simulink model "Modelo_controlador_estados"  (R2021a)
settings: Solver=FixedStepAuto  StartTime=0.0  StopTime=6  FixedStep=0.001  RelTol=1e-3
libraries: simulink x1
settings Model: Creator=faust  LastModifiedBy=franc

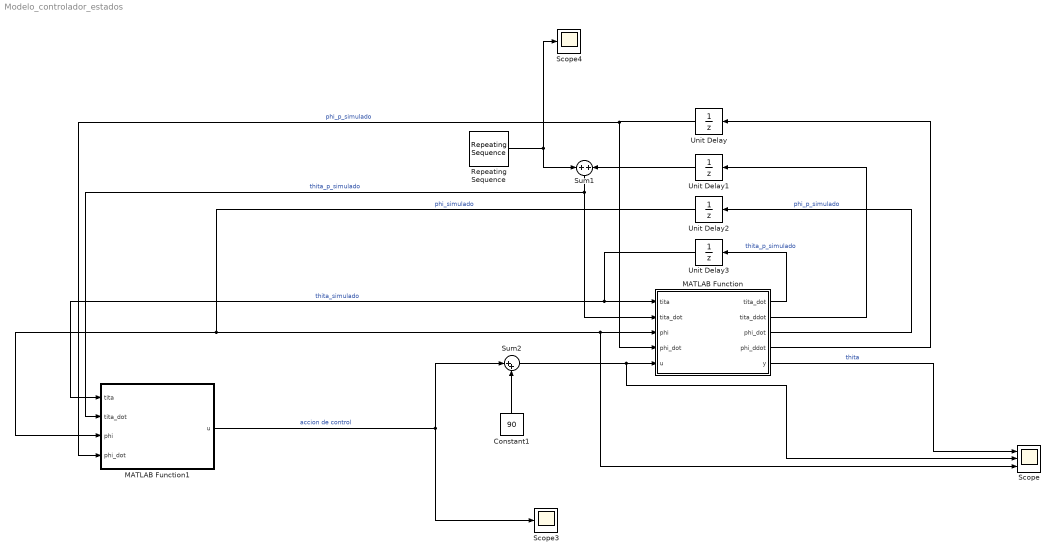
== system Modelo_controlador_estados ==
  Constant1 : Constant  Value=90
  MATLAB Function : MATLAB Function  TreatAsAtomicUnit=on
  MATLAB Function1 : MATLAB Function  TreatAsAtomicUnit=on
  Repeating Sequence : simulink/Sources/Repeating Sequence  rep_seq_t=[0 0.04 0.045 0.09 0.3 2.045 2.05 2.12 10]  rep_seq_y=[0 0 -100 0 0 0 100 0 0]
  Scope : Scope  NumInputPorts=3
  Scope3 : Scope
  Scope4 : Scope
  Sum1 : Sum  Inputs=+|+
  Sum2 : Sum  Inputs=|++
  Unit Delay : UnitDelay  SampleTime=0.01  HasFrameUpgradeWarning=on
  Unit Delay1 : UnitDelay  SampleTime=0.01  HasFrameUpgradeWarning=on
  Unit Delay2 : UnitDelay  InitialCondition=90  SampleTime=0.01  HasFrameUpgradeWarning=on
  Unit Delay3 : UnitDelay  SampleTime=0.01  HasFrameUpgradeWarning=on
  wires:
  MATLAB Function/2(tita_ddot) -> Unit Delay1/1
  Sum1/1 -> MATLAB Function1/2(tita_dot), MATLAB Function/2("tita_dot ")  "thita_p_simulado"
  MATLAB Function/5(y) -> Scope/1  "thita"
  MATLAB Function/4(phi_ddot) -> Unit Delay/1
  Unit Delay/1 -> MATLAB Function1/4(phi_dot), MATLAB Function/4("phi_dot ")  "phi_p_simulado"
  MATLAB Function/3(phi_dot) -> Unit Delay2/1  "phi_p_simulado"
  MATLAB Function1/1(u) -> Sum2/1, Scope3/1  "accion de control"
  Constant1/1 -> Sum2/2
  Unit Delay3/1 -> MATLAB Function1/1(tita), MATLAB Function/1(tita)  "thita_simulado"
  Unit Delay2/1 -> Scope/3, MATLAB Function/3(phi), MATLAB Function1/3(phi)  "phi_simulado"
  Sum2/1 -> Scope/2, MATLAB Function/5(u)
  MATLAB Function/1(tita_dot) -> Unit Delay3/1  "thita_p_simulado"
  Repeating Sequence/1 -> Scope4/1, Sum1/1
  Unit Delay1/1 -> Sum1/2

== matlab function Modelo_controlador_estados/MATLAB Function1 ==
  data: tita input; tita_dot input; u output; phi input; phi_dot input
function u = fcn(tita, tita_dot, phi, phi_dot)

K = [-0.5, 0.001, 0.7, -0.005];

phi_eq = 90;

u = K(1) * tita + K(2) * tita_dot + K(3) * (phi - phi_eq) + K(4) * phi_dot;

== matlab function Modelo_controlador_estados/MATLAB Function ==
  data: tita input; tita_dot input; tita_dot output; tita_ddot output; phi_dot output; phi input; phi_dot input; phi_ddot output; u input; y output
function [tita_dot, tita_ddot, phi_dot, phi_ddot, y] = fcn(tita, tita_dot, phi, phi_dot, u)

Ad = [
    1.0000    0.0100         0         0;
   -0.6500    0.9739   -2.0454   -0.2147;
         0         0    1.0000    0.0100;
         0         0   -2.9220    0.6933
];

Bd = [
         0;
    2.0454;
         0;
    2.9220
];

x  = [tita tita_dot phi phi_dot];
x_dot = Ad * x' + Bd * u;
tita_dot = x_dot(1);
tita_ddot = x_dot(2);
phi_dot = x_dot(3);
phi_ddot = x_dot(4);


y = x(1);
